simulink model "gm_DVBS"  (R2023b)
settings: Solver=FixedStepAuto  StartTime=0.0  StopTime=1  RelTol=1e-3
undefined symbols (not defined in the file or in its folder): alpha, fc, iniStates, rb
libraries: simulink x29, dspsrcs4 x4, commcnvcod2 x2, commsink2 x2, commdigbbndpm3 x2, commfilt2 x2, commhdlblkcod x2, hdlsllib x2, commcnvintrlv2 x1, dspsigops x1
settings Model: Creator=31651  LastModifiedBy=31651
settings SolverCC: AutoInsertRateTranBlk=on
settings OptimizationCC: BlockReduction=off  ConditionallyExecuteInputs=off  DefaultUnderspecifiedDataType=single  EnhancedBackFolding=on  PassReuseOutputArgsAs=Individual arguments  ZeroExternalMemoryAtStartup=off  ZeroInternalMemoryAtStartup=off  MaxStackSize=64  OptimizeBlockOrder=speed  DifferentSizesBufferReuse=on  OptimizationCustomize=off  EfficientTunableParamExpr=on
settings DebuggingCC: InheritedTsInSrcMsg=none  SingleTaskRateTransMsg=error  ParameterTunabilityLossMsg=error
settings HardwareCC: ProdBitPerPointer=32  ProdBitPerSizeT=32  ProdBitPerPtrDiffT=32  ProdLargestAtomicFloat=None  ProdIntDivRoundTo=Undefined  ProdEndianess=Unspecified  ProdWordSize=32  ProdHWDeviceType=ASIC/FPGA->ASIC/FPGA  TargetBitPerPointer=64  TargetBitPerSizeT=64  TargetBitPerPtrDiffT=64  TargetLongLongMode=on  TargetIntDivRoundTo=Zero  TargetEndianess=LittleEndian  TargetWordSize=64  TargetHWDeviceType=Custom Processor->MATLAB Host Computer  ProdEqTarget=off  HardwareBoardFeatureSet=SoCBlockset
settings SFSimCC: MATLABDynamicMemAlloc=off
settings RTWCC: Description=Embedded Coder  SystemTargetFile=ert.tlc  HardwareBoard=Xilinx Kintex-7 KC705 development board  TemplateMakefile=ert_default_tmf
settings CodeAppCC: ForceParamTrailComments=on  IgnoreCustomStorageClasses=off  OperatorAnnotations=on  SimulinkDataObjDesc=on  SFDataObjDesc=on  InsertBlockDesc=on

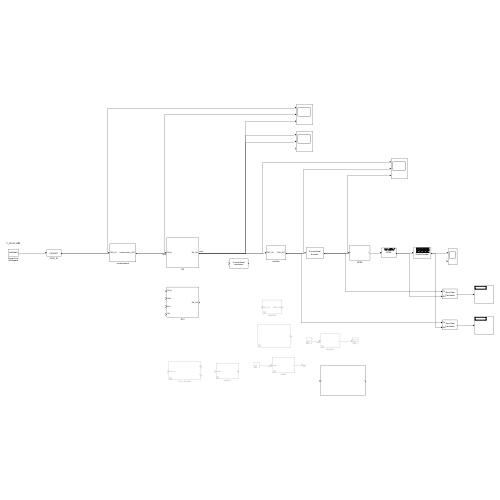
[thumbnail: Simulink's stored preview of the top-level diagram]
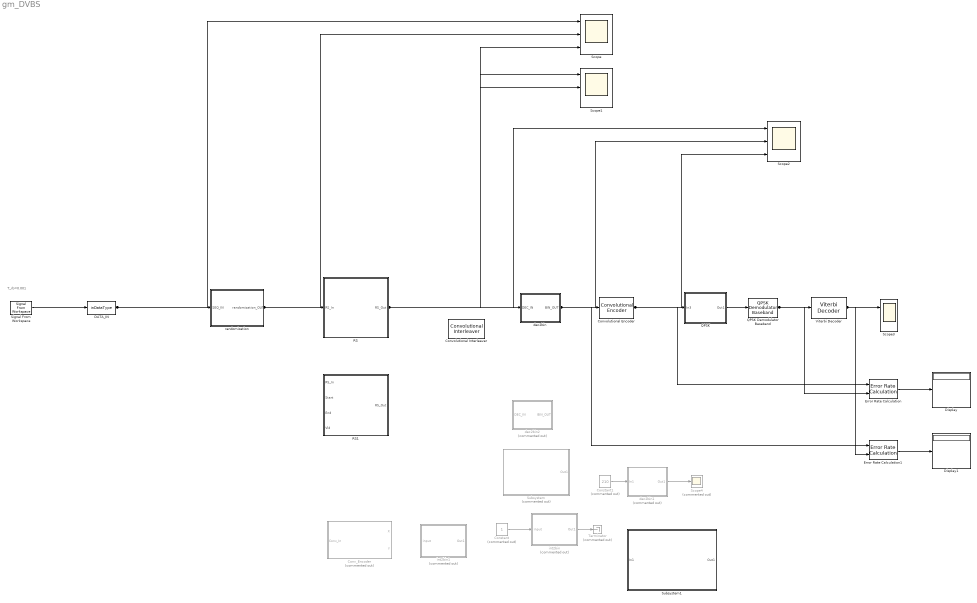
== system gm_DVBS ==
  note: T_rb=0.001
  " randomization" : Subsystem
  Constant : Constant  Commented=on  OutDataTypeStr=uint8  SampleTime=1
  Constant1 : Constant  Commented=on  Value=210  OutDataTypeStr=uint8  SampleTime=1/rb
  Conv_Encoder : Subsystem  Commented=on
  Convolutional Encoder : commcnvcod2/Convolutional Encoder  trellis=poly2trellis(7, [171 133])  opMode=Continuous  DelayedResetAction=on  hasIniStPort=off  hasFinStPort=off  usePuncVector=off  punctureVector=[1;1;0;1;1;0]  reset=Unused parameter value
      settings: LibrarySourceBlock=|
      | commhdlcnvcod/Convolutional
      | Encoder
  Convolutional Interleaver : commcnvintrlv2/Convolutional Interleaver  N=12  B=17  ic=0
      settings: LibrarySourceBlock=|
      | commhdlinterleave/Convolutional
      | Interleaver
  DATA_IN : DataTypeConversion  OutDataTypeStr=inDataType  SaturateOnIntegerOverflow=off  RndMeth=Floor
  Display : Display
  Display1 : Display
  Error Rate Calculation : commsink2/Error Rate Calculation  N=0  st_delay=0  cp_mode=Entire frame  subframe=[]  PMode=Port  WsName=ErrorVec  RsMode2=off  stop=off  numErr=100  maxBits=1e6
      settings: LibrarySourceBlock=|
      | commhdlsink/Error Rate
      | Calculation
  Error Rate Calculation1 : commsink2/Error Rate Calculation  N=64  st_delay=0  cp_mode=Entire frame  subframe=[]  PMode=Port  WsName=ErrorVec  RsMode2=off  stop=off  numErr=100  maxBits=1e6
      settings: LibrarySourceBlock=|
      | commhdlsink/Error Rate
      | Calculation
  QPSK : Subsystem
  QPSK Demodulator Baseband : commdigbbndpm3/QPSK Demodulator Baseband  OutType=Bit  DecType=Hard decision  VarSource=Dialog  Variance=1  Dec=Binary  Ph=pi/4  outDtype1=double  outDtype2=Inherit via internal rule  derotateFactorWordLen=16  derotateFactorDataTypeStr=Inherit: Same word length as input  derotateFactorLastDataTypeStr=Inherit: Same word length as input
      settings: LibrarySourceBlock=|
      | commhdldigbbndpm/QPSK
      | Demodulator
      | Baseband
  RS : Subsystem
  RS1 : Subsystem
  Scope : Scope  NumInputPorts=3
  Scope1 : Scope  NumInputPorts=3
  Scope2 : Scope  NumInputPorts=3
  Scope3 : Scope  NumInputPorts=2
  Scope4 : Scope  Commented=on
  Signal From Workspace : dspsrcs4/Signal From Workspace  X=simDataIn  Ts=1/rb  nsamps=1  OutputAfterFinalValue=Setting to zero  ignoreOrWarnInputAndFrameLengths=off  OutputFrames=off
  Subsystem : Subsystem  Commented=on
  Subsystem1 : Subsystem
  Terminator : Terminator  Commented=on
  Viterbi Decoder : commcnvcod2/Viterbi Decoder  trellis=poly2trellis(7, [171 133])  isPunctured=off  punctureVector=[1; 1; 0; 1; 0; 1]  erasures=off  dectype=Unquantized  nsdecb=4  runSigValErrCheck=off  tbdepth=64  opmode=Continuous  reset=off  delayedResetAction=off  smWordLength=16  outDataType=Inherit via internal rule
  dec2bin : Subsystem
  dec2bin1 : Subsystem  Commented=on
  dec2bin2 : Subsystem  Commented=on
  int2bin : Subsystem  Commented=on
  int2bin1 : Subsystem  Commented=on
  wires:
  Error Rate Calculation1/1 -> Display1/1
  Error Rate Calculation/1 -> Display/1
  QPSK Demodulator Baseband/1 -> Viterbi Decoder/1, Error Rate Calculation/2
  dec2bin/1(BIN_OUT) -> Scope2/2, Convolutional Encoder/1, Error Rate Calculation1/1
  QPSK/1(Out1) -> QPSK Demodulator Baseband/1
  RS/1(RS_Out) -> Scope1/1, dec2bin/1(DEC_IN), Scope1/2, Scope2/1, Scope/3
  dec2bin1/1(Out1) -> Scope4/1
  Constant1/1 -> dec2bin1/1(In1)
  Viterbi Decoder/1 -> Scope3/1, Error Rate Calculation1/2
  Convolutional Encoder/1 -> Scope2/3, QPSK/1(In3), Error Rate Calculation/1
  int2bin/1(Out1) -> Terminator/1
  Constant/1 -> int2bin/1(input)
  Signal From Workspace/1 -> DATA_IN/1
  " randomization"/1(" randomization_OUT") -> Scope/2, RS/1(RS_In)
  DATA_IN/1 -> Scope/1, " randomization"/1(SEQ_IN)

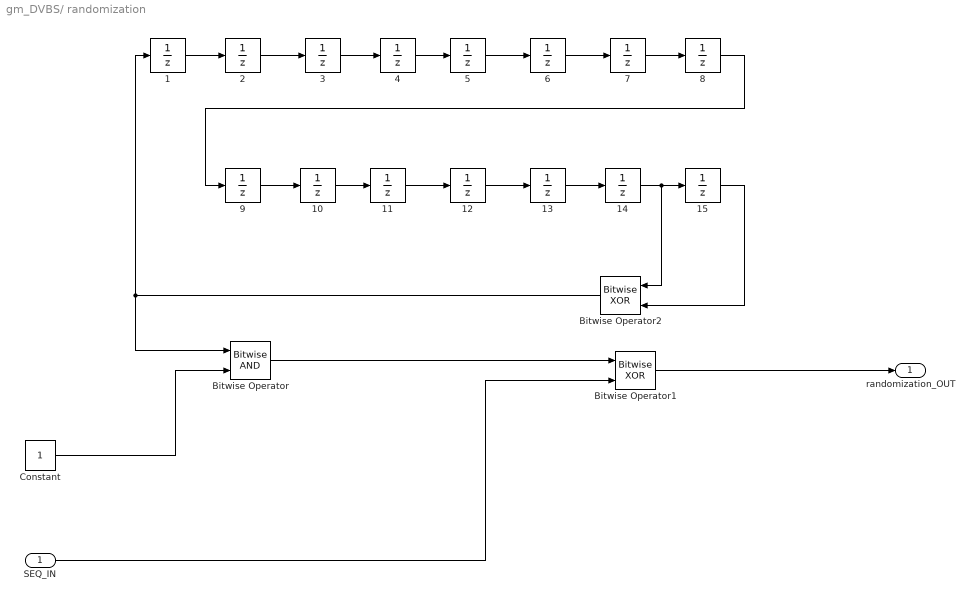
== system gm_DVBS/ randomization ==
  SEQ_IN : Inport
  1 : UnitDelay  InitialCondition=iniStates(1)  SampleTime=1/rb  HasFrameUpgradeWarning=on
  10 : UnitDelay  InitialCondition=iniStates(10)  SampleTime=-1  HasFrameUpgradeWarning=on
  11 : UnitDelay  InitialCondition=iniStates(11)  SampleTime=-1  HasFrameUpgradeWarning=on
  12 : UnitDelay  InitialCondition=iniStates(12)  SampleTime=-1  HasFrameUpgradeWarning=on
  13 : UnitDelay  InitialCondition=iniStates(13)  SampleTime=-1  HasFrameUpgradeWarning=on
  14 : UnitDelay  InitialCondition=iniStates(14)  SampleTime=-1  HasFrameUpgradeWarning=on
  15 : UnitDelay  InitialCondition=iniStates(15)  SampleTime=-1  HasFrameUpgradeWarning=on
  2 : UnitDelay  InitialCondition=iniStates(2)  SampleTime=-1  HasFrameUpgradeWarning=on
  3 : UnitDelay  InitialCondition=iniStates(3)  SampleTime=-1  HasFrameUpgradeWarning=on
  4 : UnitDelay  InitialCondition=iniStates(4)  SampleTime=-1  HasFrameUpgradeWarning=on
  5 : UnitDelay  InitialCondition=iniStates(5)  SampleTime=-1  HasFrameUpgradeWarning=on
  6 : UnitDelay  InitialCondition=iniStates(6)  SampleTime=-1  HasFrameUpgradeWarning=on
  7 : UnitDelay  InitialCondition=iniStates(7)  SampleTime=-1  HasFrameUpgradeWarning=on
  8 : UnitDelay  InitialCondition=iniStates(8)  SampleTime=-1  HasFrameUpgradeWarning=on
  9 : UnitDelay  InitialCondition=iniStates(9)  SampleTime=-1  HasFrameUpgradeWarning=on
  Bitwise Operator : simulink/Logic and Bit Operations/Bitwise Operator  logicop=AND  UseBitMask=off  NumInputPorts=2  BitMask=bin2dec('11011001')  BitMaskRealWorld=Stored Integer
      settings: LibrarySourceBlock=|
      | hdlsllib/Logic and Bit
      | Operations/Bitwise
      | Operator
  Bitwise Operator1 : simulink/Logic and Bit Operations/Bitwise Operator  logicop=XOR  UseBitMask=off  NumInputPorts=2  BitMask=bin2dec('11011001')  BitMaskRealWorld=Stored Integer
      settings: LibrarySourceBlock=|
      | hdlsllib/Logic and Bit
      | Operations/Bitwise
      | Operator
  Bitwise Operator2 : simulink/Logic and Bit Operations/Bitwise Operator  logicop=XOR  UseBitMask=off  NumInputPorts=2  BitMask=bin2dec('11011001')  BitMaskRealWorld=Stored Integer
      settings: LibrarySourceBlock=|
      | hdlsllib/Logic and Bit
      | Operations/Bitwise
      | Operator
  Constant : Constant  OutDataTypeStr=inDataType  SampleTime=1/rb
  " randomization_OUT" : Outport
  wires:
  Bitwise Operator1/1 -> " randomization_OUT"/1
  SEQ_IN/1 -> Bitwise Operator1/2
  Constant/1 -> Bitwise Operator/2
  Bitwise Operator/1 -> Bitwise Operator1/1
  Bitwise Operator2/1 -> 1/1, Bitwise Operator/1
  15/1 -> Bitwise Operator2/2
  12/1 -> 13/1
  13/1 -> 14/1
  14/1 -> 15/1, Bitwise Operator2/1
  6/1 -> 7/1
  7/1 -> 8/1
  11/1 -> 12/1
  8/1 -> 9/1
  10/1 -> 11/1
  9/1 -> 10/1
  1/1 -> 2/1
  3/1 -> 4/1
  2/1 -> 3/1
  4/1 -> 5/1
  5/1 -> 6/1

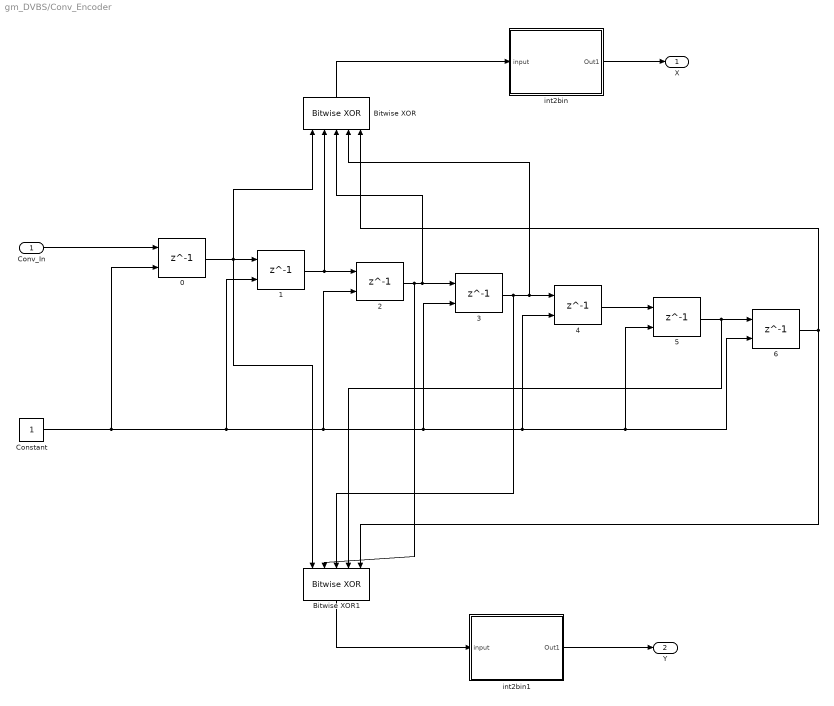
== system gm_DVBS/Conv_Encoder ==
  Conv_In : Inport
  {0..6} (7 alike) : Delay  DelayLength=1  ShowEnablePort=on
      settings: InputPortMap=u0,e6
  Bitwise XOR : simulink/Logic and Bit Operations/Bitwise Operator  logicop=XOR  UseBitMask=off  NumInputPorts=5  BitMask=bin2dec('11011001')  BitMaskRealWorld=Stored Integer
      settings: LibrarySourceBlock=|
      | simulink/Quick Insert/Logic and Bit
      | Operations/Bitwise XOR
  Bitwise XOR1 : simulink/Logic and Bit Operations/Bitwise Operator  logicop=XOR  UseBitMask=off  NumInputPorts=5  BitMask=bin2dec('11011001')  BitMaskRealWorld=Stored Integer
      settings: LibrarySourceBlock=|
      | simulink/Quick Insert/Logic and Bit
      | Operations/Bitwise XOR
  Constant : Constant  OutDataTypeStr=boolean  SampleTime=1/rb
  int2bin : Subsystem
  int2bin1 : Subsystem
  X : Outport
  Y : Outport  Port=2
  wires:
  int2bin1/1(Out1) -> Y/1
  Bitwise XOR/1 -> int2bin/1(input)
  int2bin/1(Out1) -> X/1
  Bitwise XOR1/1 -> int2bin1/1(input)
  6/1 -> Bitwise XOR/5, Bitwise XOR1/5
  Constant/1 -> 6/2, 5/2, 4/2, 3/2, 2/2, 1/2, 0/2
  Conv_In/1 -> 0/1
  0/1 -> 1/1, Bitwise XOR/1, Bitwise XOR1/1
  1/1 -> 2/1, Bitwise XOR/2
  2/1 -> 3/1, Bitwise XOR/3, Bitwise XOR1/2
  3/1 -> 4/1, Bitwise XOR/4, Bitwise XOR1/3
  4/1 -> 5/1
  5/1 -> 6/1, Bitwise XOR1/4

== system gm_DVBS/QPSK ==
  In3 : Inport
  Add : Sum
  Complex to Real-Imag : ComplexToRealImag
  Cos : Sin  Frequency=fc*2*pi  Phase=pi/2  SampleTime=0
  Product : Product
  Product1 : Product
  QPSK Modulator Baseband : commdigbbndpm3/QPSK Modulator Baseband  InType=Bit  Enc=Binary  Ph=pi/4  outDtype=double  outWordLen=16  outUDDataType=sfix(16)  outFracLenMode=Best precision  outFracLen=15  outDataTypeStr=double  outLastDataTypeStr=double
      settings: LibrarySourceBlock=|
      | commhdldigbbndpm/QPSK
      | Modulator
      | Baseband
  Raised Cosine Transmit Filter2 : commfilt2/Raised Cosine Transmit Filter  filtType=Square root  R=alpha  filtSpan=10  N=8  filterGain=1  InputProcessing=Columns as channels (frame based)  RateOptions=Allow multirate processing  framing=Mute  checkCoeff=off  variableName=rcTxFilt2  checkGain=Normalized  sampMode=Mute  saveAsFlag=0  currentFiltSpan=10  D=5  launchFVT=on  roundingMode=Floor  overflowMode=off  coeffDataTypeStr=Inherit: Same word length as input  coeffMin=[]  coeffMax=[]  coeffLastDataTypeStr=Inherit: Same word length as input  outputDataTypeStr=Inherit: Same as accumulator  outputMin=[]  outputMax=[]  outputLastDataTypeStr=Inherit: Same as accumulator
      settings: LibrarySourceBlock=|
      | commhdlfilt/Raised Cosine
      | Transmit Filter
  Raised Cosine Transmit Filter3 : commfilt2/Raised Cosine Transmit Filter  filtType=Square root  R=alpha  filtSpan=10  N=8  filterGain=1  RateOptions=Allow multirate processing  framing=Mute  checkCoeff=off  variableName=rcTxFilt3  checkGain=Normalized  sampMode=Mute  saveAsFlag=0  currentFiltSpan=10  D=5  launchFVT=on  roundingMode=Floor  overflowMode=off  coeffDataTypeStr=Inherit: Same word length as input  coeffMin=[]  coeffMax=[]  coeffLastDataTypeStr=Inherit: Same word length as input  outputDataTypeStr=Inherit: Same as accumulator  outputMin=[]  outputMax=[]  outputLastDataTypeStr=Inherit: Same as accumulator
      settings: LibrarySourceBlock=|
      | commhdlfilt/Raised Cosine
      | Transmit Filter
  Scope : Scope
  Scope1 : Scope  NumInputPorts=2
  Sin : Sin  Frequency=fc*2*pi  SampleTime=0
  Spectrum Analyzer : SpectrumAnalyzer  WindowPosition=[560.000000,290.000000,800.000000,500.000000,]  ScopeFrameLocation=window  Span=24000  StartFrequency=-12000  StopFrequency=12000  YLimits=[-206.50491474,-40.69069962]
      settings: OpenAtSimulationStart=off
  Zero-Order Hold : ZeroOrderHold  SampleTime=-1
  Out1 : Outport
  wires:
  Zero-Order Hold/1 -> Spectrum Analyzer/1
  Add/1 -> Zero-Order Hold/1, Scope/1
  Product1/1 -> Add/2
  Complex to Real-Imag/2 -> Raised Cosine Transmit Filter3/1
  Cos/1 -> Product/2, Scope1/2
  Sin/1 -> Product1/1
  Complex to Real-Imag/1 -> Raised Cosine Transmit Filter2/1
  Raised Cosine Transmit Filter2/1 -> Product/1
  Raised Cosine Transmit Filter3/1 -> Product1/2
  Product/1 -> Add/1, Scope1/1
  In3/1 -> QPSK Modulator Baseband/1
  QPSK Modulator Baseband/1 -> Complex to Real-Imag/1, Out1/1

== system gm_DVBS/RS ==
  RS_In : Inport  OutDataTypeStr=uint8
  Data Type Conversion : DataTypeConversion  OutDataTypeStr=boolean  SaturateOnIntegerOverflow=off  RndMeth=Floor
  Data Type Conversion1 : DataTypeConversion  OutDataTypeStr=boolean  SaturateOnIntegerOverflow=off  RndMeth=Floor
  Data Type Conversion2 : DataTypeConversion  OutDataTypeStr=boolean  SaturateOnIntegerOverflow=off  RndMeth=Floor
  Integer-Input RS Encoder HDL Optimized : commhdlblkcod/Integer-Input RS Encoder HDL Optimized  CodewordLength=n  MessageLength=k  PrimitivePolynomialSource=Auto  PrimitivePolynomial=[ 1, 0, 1, 1 ]  PuncturePatternSource=None  PuncturePattern=[ ones( 2, 1 ); zeros( 2, 1 ) ]  BSource=Auto  B=1  SimulateUsing=Code generation
  Signal From Workspace1 : dspsrcs4/Signal From Workspace  X=simStart  Ts=1/rb  nsamps=1  OutputAfterFinalValue=Setting to zero  ignoreOrWarnInputAndFrameLengths=off  OutputFrames=off
  Signal From Workspace2 : dspsrcs4/Signal From Workspace  X=simEnd  Ts=1/rb  nsamps=1  OutputAfterFinalValue=Setting to zero  ignoreOrWarnInputAndFrameLengths=off  OutputFrames=off
  Signal From Workspace3 : dspsrcs4/Signal From Workspace  X=simValidIn  Ts=1/rb  nsamps=1  OutputAfterFinalValue=Setting to zero  ignoreOrWarnInputAndFrameLengths=off  OutputFrames=off
  RS_Out : Outport  OutDataTypeStr=uint8
  wires:
  Integer-Input RS Encoder HDL Optimized/1 -> RS_Out/1
  RS_In/1 -> Integer-Input RS Encoder HDL Optimized/1
  Data Type Conversion2/1 -> Integer-Input RS Encoder HDL Optimized/4
  Signal From Workspace1/1 -> Data Type Conversion/1
  Signal From Workspace2/1 -> Data Type Conversion1/1
  Signal From Workspace3/1 -> Data Type Conversion2/1
  Data Type Conversion1/1 -> Integer-Input RS Encoder HDL Optimized/3
  Data Type Conversion/1 -> Integer-Input RS Encoder HDL Optimized/2

== system gm_DVBS/RS1 ==
  RS_In : Inport  OutDataTypeStr=uint8
  Start : Inport  Port=2
  End : Inport  Port=3
  Vld : Inport  Port=4
  Data Type Conversion : DataTypeConversion  OutDataTypeStr=boolean  SaturateOnIntegerOverflow=off  RndMeth=Floor
  Data Type Conversion1 : DataTypeConversion  OutDataTypeStr=boolean  SaturateOnIntegerOverflow=off  RndMeth=Floor
  Data Type Conversion2 : DataTypeConversion  OutDataTypeStr=boolean  SaturateOnIntegerOverflow=off  RndMeth=Floor
  Integer-Input RS Encoder HDL Optimized : commhdlblkcod/Integer-Input RS Encoder HDL Optimized  CodewordLength=n  MessageLength=k  PrimitivePolynomialSource=Auto  PrimitivePolynomial=[ 1, 0, 1, 1 ]  PuncturePatternSource=None  PuncturePattern=[ ones( 2, 1 ); zeros( 2, 1 ) ]  BSource=Auto  B=1  SimulateUsing=Code generation
  Terminator : Terminator
  Terminator1 : Terminator
  Terminator2 : Terminator
  RS_Out : Outport  OutDataTypeStr=uint8
  wires:
  Integer-Input RS Encoder HDL Optimized/4 -> Terminator2/1
  Integer-Input RS Encoder HDL Optimized/3 -> Terminator1/1
  Integer-Input RS Encoder HDL Optimized/2 -> Terminator/1
  Vld/1 -> Data Type Conversion2/1
  End/1 -> Data Type Conversion1/1
  Start/1 -> Data Type Conversion/1
  Integer-Input RS Encoder HDL Optimized/1 -> RS_Out/1
  RS_In/1 -> Integer-Input RS Encoder HDL Optimized/1
  Data Type Conversion2/1 -> Integer-Input RS Encoder HDL Optimized/4
  Data Type Conversion1/1 -> Integer-Input RS Encoder HDL Optimized/3
  Data Type Conversion/1 -> Integer-Input RS Encoder HDL Optimized/2

== system gm_DVBS/Subsystem ==
  Constant1 : Constant  Value=113  SampleTime=1
  Demux : Demux  Outputs=8
      settings: DisplayOption=none
  MATLAB Function : MATLAB Function  TreatAsAtomicUnit=on
  Scope : Scope
  Subsystem1 : Subsystem
  Out1 : Outport
  wires:
  Subsystem1/1(Out1) -> Out1/1, Scope/1
  MATLAB Function/1(bin_out) -> Demux/1
  Demux/8 -> Subsystem1/8(In8)
  Demux/7 -> Subsystem1/7(In7)
  Demux/6 -> Subsystem1/6(In6)
  Demux/5 -> Subsystem1/5(In5)
  Demux/4 -> Subsystem1/4(In4)
  Demux/3 -> Subsystem1/3(In3)
  Demux/2 -> Subsystem1/2(In2)
  Demux/1 -> Subsystem1/1(In1)
  Constant1/1 -> MATLAB Function/1(dec_in)

== system gm_DVBS/Subsystem1 ==
  In1 : Inport
  Out1 : Outport
  wires:
  In1/1 -> Out1/1

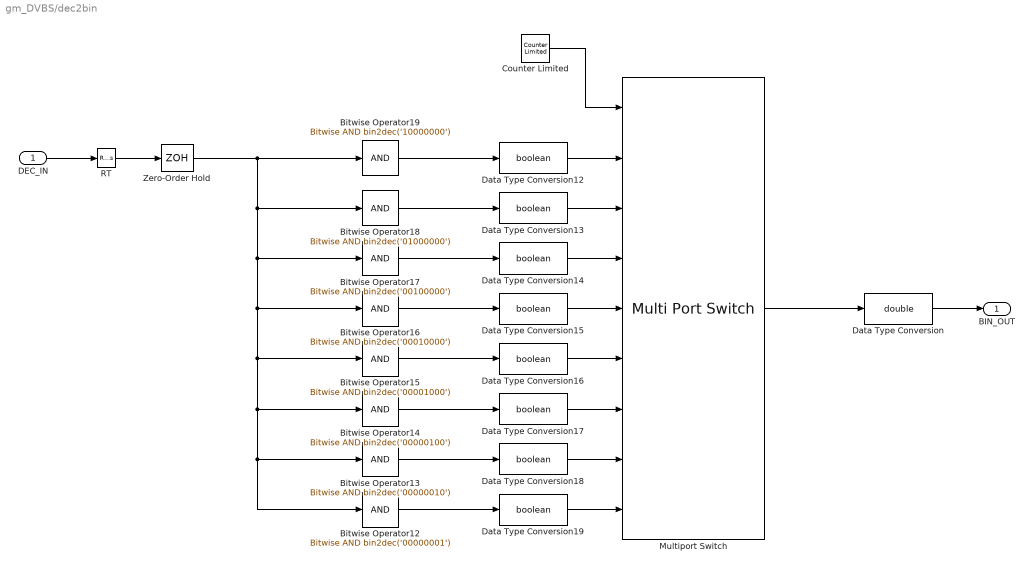
== system gm_DVBS/dec2bin ==
  DEC_IN : Inport
  Bitwise Operator12 : simulink/Logic and Bit Operations/Bitwise Operator  logicop=AND  UseBitMask=on  BitMask=bin2dec('00000001')  BitMaskRealWorld=Stored Integer
  Bitwise Operator13 : simulink/Logic and Bit Operations/Bitwise Operator  logicop=AND  UseBitMask=on  BitMask=bin2dec('00000010')  BitMaskRealWorld=Stored Integer
  Bitwise Operator14 : simulink/Logic and Bit Operations/Bitwise Operator  logicop=AND  UseBitMask=on  BitMask=bin2dec('00000100')  BitMaskRealWorld=Stored Integer
  Bitwise Operator15 : simulink/Logic and Bit Operations/Bitwise Operator  logicop=AND  UseBitMask=on  BitMask=bin2dec('00001000')  BitMaskRealWorld=Stored Integer
  Bitwise Operator16 : simulink/Logic and Bit Operations/Bitwise Operator  logicop=AND  UseBitMask=on  BitMask=bin2dec('00010000')  BitMaskRealWorld=Stored Integer
  Bitwise Operator17 : simulink/Logic and Bit Operations/Bitwise Operator  logicop=AND  UseBitMask=on  BitMask=bin2dec('00100000')  BitMaskRealWorld=Stored Integer
  Bitwise Operator18 : simulink/Logic and Bit Operations/Bitwise Operator  logicop=AND  UseBitMask=on  BitMask=bin2dec('01000000')  BitMaskRealWorld=Stored Integer
  Bitwise Operator19 : simulink/Logic and Bit Operations/Bitwise Operator  logicop=AND  UseBitMask=on  BitMask=bin2dec('10000000')  BitMaskRealWorld=Stored Integer
  Counter Limited : hdlsllib/Sources/Counter Limited  uplimit=7  tsamp=0.125/rb
  Data Type Conversion : DataTypeConversion  OutDataTypeStr=double  SaturateOnIntegerOverflow=off  RndMeth=Floor
  Data Type Conversion{12..19} (8 alike) : DataTypeConversion  OutDataTypeStr=boolean  SaturateOnIntegerOverflow=off  RndMeth=Floor
  Multiport Switch : MultiPortSwitch  DataPortOrder=Zero-based contiguous  Inputs=8  zeroidx=on  SaturateOnIntegerOverflow=off  InputSameDT=off
  RT : RateTransition  OutPortSampleTime=0.000125
  Zero-Order Hold : ZeroOrderHold  SampleTime=0.125/rb
  BIN_OUT : Outport
  wires:
  Data Type Conversion/1 -> BIN_OUT/1
  Multiport Switch/1 -> Data Type Conversion/1
  RT/1 -> Zero-Order Hold/1
  Zero-Order Hold/1 -> Bitwise Operator17/1, Bitwise Operator14/1, Bitwise Operator12/1, Bitwise Operator13/1, Bitwise Operator15/1, Bitwise Operator16/1, Bitwise Operator18/1, Bitwise Operator19/1
  Bitwise Operator17/1 -> Data Type Conversion14/1
  Data Type Conversion19/1 -> Multiport Switch/9
  Data Type Conversion17/1 -> Multiport Switch/7
  Data Type Conversion13/1 -> Multiport Switch/3
  Bitwise Operator12/1 -> Data Type Conversion19/1
  Data Type Conversion16/1 -> Multiport Switch/6
  Data Type Conversion15/1 -> Multiport Switch/5
  Data Type Conversion14/1 -> Multiport Switch/4
  Data Type Conversion18/1 -> Multiport Switch/8
  Data Type Conversion12/1 -> Multiport Switch/2
  Bitwise Operator16/1 -> Data Type Conversion15/1
  Counter Limited/1 -> Multiport Switch/1
  DEC_IN/1 -> RT/1
  Bitwise Operator14/1 -> Data Type Conversion17/1
  Bitwise Operator15/1 -> Data Type Conversion16/1
  Bitwise Operator19/1 -> Data Type Conversion12/1
  Bitwise Operator18/1 -> Data Type Conversion13/1
  Bitwise Operator13/1 -> Data Type Conversion18/1

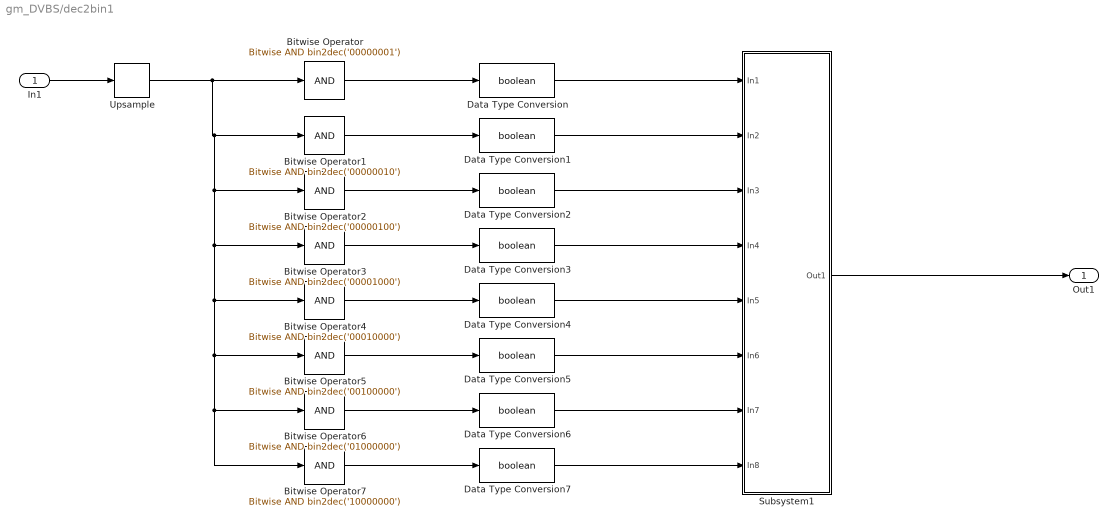
== system gm_DVBS/dec2bin1 ==
  In1 : Inport  OutDataTypeStr=uint8
  Bitwise Operator : simulink/Logic and Bit Operations/Bitwise Operator  logicop=AND  UseBitMask=on  BitMask=bin2dec('00000001')  BitMaskRealWorld=Stored Integer
  Bitwise Operator1 : simulink/Logic and Bit Operations/Bitwise Operator  logicop=AND  UseBitMask=on  BitMask=bin2dec('00000010')  BitMaskRealWorld=Stored Integer
  Bitwise Operator2 : simulink/Logic and Bit Operations/Bitwise Operator  logicop=AND  UseBitMask=on  BitMask=bin2dec('00000100')  BitMaskRealWorld=Stored Integer
  Bitwise Operator3 : simulink/Logic and Bit Operations/Bitwise Operator  logicop=AND  UseBitMask=on  BitMask=bin2dec('00001000')  BitMaskRealWorld=Stored Integer
  Bitwise Operator4 : simulink/Logic and Bit Operations/Bitwise Operator  logicop=AND  UseBitMask=on  BitMask=bin2dec('00010000')  BitMaskRealWorld=Stored Integer
  Bitwise Operator5 : simulink/Logic and Bit Operations/Bitwise Operator  logicop=AND  UseBitMask=on  BitMask=bin2dec('00100000')  BitMaskRealWorld=Stored Integer
  Bitwise Operator6 : simulink/Logic and Bit Operations/Bitwise Operator  logicop=AND  UseBitMask=on  BitMask=bin2dec('01000000')  BitMaskRealWorld=Stored Integer
  Bitwise Operator7 : simulink/Logic and Bit Operations/Bitwise Operator  logicop=AND  UseBitMask=on  BitMask=bin2dec('10000000')  BitMaskRealWorld=Stored Integer
  Data Type Conversion{,1..7} (8 alike) : DataTypeConversion  OutDataTypeStr=boolean  SaturateOnIntegerOverflow=off  RndMeth=Floor
  Subsystem1 : Subsystem
  Upsample : dspsigops/Upsample  FactorSource=Dialog parameter  N=3  Nmax=16  phase=0  RateOptions=Allow multirate processing  ic=0  mode=Unused parameter value
      settings: LibrarySourceBlock=dsphdlsupportsigops/Upsample
  Out1 : Outport
  wires:
  Upsample/1 -> Bitwise Operator/1, Bitwise Operator1/1, Bitwise Operator2/1, Bitwise Operator3/1, Bitwise Operator4/1, Bitwise Operator5/1, Bitwise Operator6/1, Bitwise Operator7/1
  Bitwise Operator/1 -> Data Type Conversion/1
  Bitwise Operator1/1 -> Data Type Conversion1/1
  Bitwise Operator3/1 -> Data Type Conversion3/1
  Bitwise Operator4/1 -> Data Type Conversion4/1
  Bitwise Operator2/1 -> Data Type Conversion2/1
  Data Type Conversion2/1 -> Subsystem1/3(In3)
  Bitwise Operator5/1 -> Data Type Conversion5/1
  Bitwise Operator6/1 -> Data Type Conversion6/1
  Bitwise Operator7/1 -> Data Type Conversion7/1
  In1/1 -> Upsample/1
  Data Type Conversion3/1 -> Subsystem1/4(In4)
  Subsystem1/1(Out1) -> Out1/1
  Data Type Conversion6/1 -> Subsystem1/7(In7)
  Data Type Conversion1/1 -> Subsystem1/2(In2)
  Data Type Conversion7/1 -> Subsystem1/8(In8)
  Data Type Conversion5/1 -> Subsystem1/6(In6)
  Data Type Conversion/1 -> Subsystem1/1(In1)
  Data Type Conversion4/1 -> Subsystem1/5(In5)

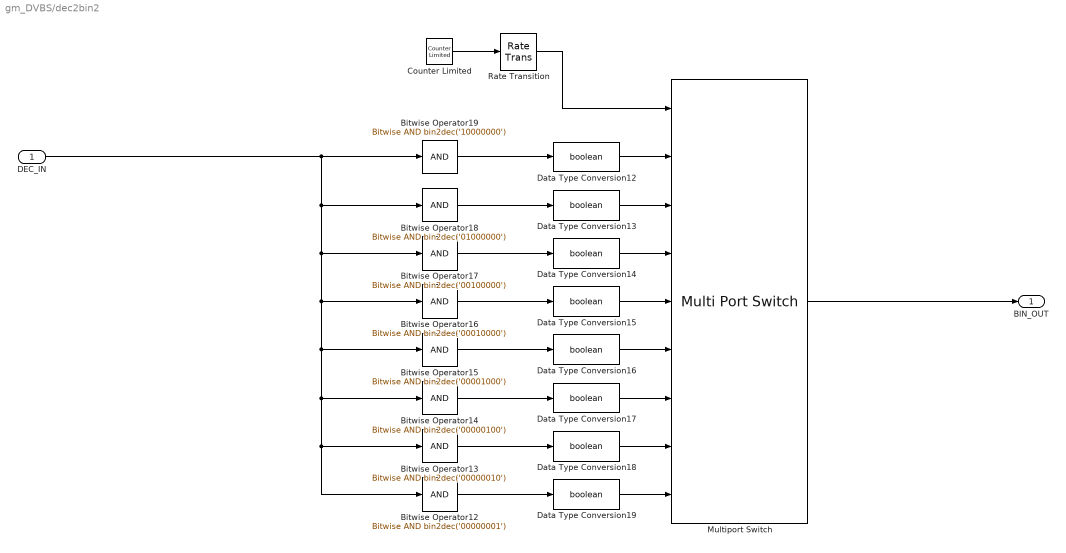
== system gm_DVBS/dec2bin2 ==
  DEC_IN : Inport  OutDataTypeStr=uint8
  Bitwise Operator12 : simulink/Logic and Bit Operations/Bitwise Operator  logicop=AND  UseBitMask=on  BitMask=bin2dec('00000001')  BitMaskRealWorld=Stored Integer
  Bitwise Operator13 : simulink/Logic and Bit Operations/Bitwise Operator  logicop=AND  UseBitMask=on  BitMask=bin2dec('00000010')  BitMaskRealWorld=Stored Integer
  Bitwise Operator14 : simulink/Logic and Bit Operations/Bitwise Operator  logicop=AND  UseBitMask=on  BitMask=bin2dec('00000100')  BitMaskRealWorld=Stored Integer
  Bitwise Operator15 : simulink/Logic and Bit Operations/Bitwise Operator  logicop=AND  UseBitMask=on  BitMask=bin2dec('00001000')  BitMaskRealWorld=Stored Integer
  Bitwise Operator16 : simulink/Logic and Bit Operations/Bitwise Operator  logicop=AND  UseBitMask=on  BitMask=bin2dec('00010000')  BitMaskRealWorld=Stored Integer
  Bitwise Operator17 : simulink/Logic and Bit Operations/Bitwise Operator  logicop=AND  UseBitMask=on  BitMask=bin2dec('00100000')  BitMaskRealWorld=Stored Integer
  Bitwise Operator18 : simulink/Logic and Bit Operations/Bitwise Operator  logicop=AND  UseBitMask=on  BitMask=bin2dec('01000000')  BitMaskRealWorld=Stored Integer
  Bitwise Operator19 : simulink/Logic and Bit Operations/Bitwise Operator  logicop=AND  UseBitMask=on  BitMask=bin2dec('10000000')  BitMaskRealWorld=Stored Integer
  Counter Limited : hdlsllib/Sources/Counter Limited  uplimit=7  tsamp=0.125/rb
  Data Type Conversion{12..19} (8 alike) : DataTypeConversion  OutDataTypeStr=boolean  SaturateOnIntegerOverflow=off  RndMeth=Floor
  Multiport Switch : MultiPortSwitch  DataPortOrder=Zero-based contiguous  Inputs=8  zeroidx=on  SaturateOnIntegerOverflow=off  InputSameDT=off
  Rate Transition : RateTransition  OutPortSampleTime=0.125/rb
  BIN_OUT : Outport
  wires:
  Rate Transition/1 -> Multiport Switch/1
  DEC_IN/1 -> Bitwise Operator19/1, Bitwise Operator17/1, Bitwise Operator14/1, Bitwise Operator12/1, Bitwise Operator13/1, Bitwise Operator15/1, Bitwise Operator16/1, Bitwise Operator18/1
  Counter Limited/1 -> Rate Transition/1
  Multiport Switch/1 -> BIN_OUT/1
  Bitwise Operator17/1 -> Data Type Conversion14/1
  Data Type Conversion19/1 -> Multiport Switch/9
  Data Type Conversion17/1 -> Multiport Switch/7
  Data Type Conversion13/1 -> Multiport Switch/3
  Bitwise Operator12/1 -> Data Type Conversion19/1
  Data Type Conversion16/1 -> Multiport Switch/6
  Data Type Conversion15/1 -> Multiport Switch/5
  Data Type Conversion14/1 -> Multiport Switch/4
  Data Type Conversion18/1 -> Multiport Switch/8
  Data Type Conversion12/1 -> Multiport Switch/2
  Bitwise Operator16/1 -> Data Type Conversion15/1
  Bitwise Operator14/1 -> Data Type Conversion17/1
  Bitwise Operator15/1 -> Data Type Conversion16/1
  Bitwise Operator19/1 -> Data Type Conversion12/1
  Bitwise Operator18/1 -> Data Type Conversion13/1
  Bitwise Operator13/1 -> Data Type Conversion18/1

== system gm_DVBS/int2bin ==
  note: 最低位
  input : Inport  OutDataTypeStr=uint8
  Data Type Conversion : DataTypeConversion  OutDataTypeStr=boolean  SaturateOnIntegerOverflow=off  RndMeth=Floor
  Demux : Demux  Outputs=8
      settings: DisplayOption=none
  PISO : Subsystem
  Scope3 : Scope  NumInputPorts=4
  Scope4 : Scope  NumInputPorts=4
  uint8tobin : MATLAB Function  TreatAsAtomicUnit=on
  Out1 : Outport
  wires:
  Data Type Conversion/1 -> Demux/1
  Demux/2 -> Scope3/2, PISO/2(2)
  Demux/3 -> Scope3/3, PISO/3(3)
  Demux/4 -> Scope3/4, PISO/4(4)
  input/1 -> uint8tobin/1(input)
  Demux/7 -> Scope4/3, PISO/7(7)
  Demux/1 -> Scope3/1, PISO/1(1)
  uint8tobin/1(bitValue) -> Data Type Conversion/1
  Demux/8 -> Scope4/4, PISO/8(8)
  Demux/5 -> Scope4/1, PISO/5(5)
  Demux/6 -> Scope4/2, PISO/6(6)
  PISO/1(Out1) -> Out1/1

== system gm_DVBS/int2bin1 ==
  note: 最低位
  input : Inport  OutDataTypeStr=uint8
  Data Type Conversion : DataTypeConversion  OutDataTypeStr=boolean  SaturateOnIntegerOverflow=off  RndMeth=Floor
  Demux : Demux  Outputs=8
      settings: DisplayOption=none
  PISO : Subsystem
  Scope3 : Scope  NumInputPorts=4
  Scope4 : Scope  NumInputPorts=4
  uint8tobin : MATLAB Function  TreatAsAtomicUnit=on
  Out1 : Outport
  wires:
  Data Type Conversion/1 -> Demux/1
  Demux/2 -> Scope3/2, PISO/2(2)
  Demux/3 -> Scope3/3, PISO/3(3)
  Demux/4 -> Scope3/4, PISO/4(4)
  input/1 -> uint8tobin/1(input)
  Demux/7 -> Scope4/3, PISO/7(7)
  Demux/1 -> Scope3/1, PISO/1(1)
  uint8tobin/1(bitValue) -> Data Type Conversion/1
  Demux/8 -> Scope4/4, PISO/8(8)
  Demux/5 -> Scope4/1, PISO/5(5)
  Demux/6 -> Scope4/2, PISO/6(6)
  PISO/1(Out1) -> Out1/1

== system gm_DVBS/Conv_Encoder/int2bin ==
  note: 最低位
  input : Inport
  Demux : Demux  Outputs=8
      settings: DisplayOption=none
  PISO : Subsystem
  Scope3 : Scope  NumInputPorts=4
  Scope4 : Scope  NumInputPorts=4
  uint8tobin : MATLAB Function  TreatAsAtomicUnit=on
  Out1 : Outport
  wires:
  Demux/2 -> Scope3/2, PISO/2(2)
  Demux/3 -> Scope3/3, PISO/3(3)
  Demux/4 -> Scope3/4, PISO/4(4)
  input/1 -> uint8tobin/1(input)
  Demux/7 -> Scope4/3, PISO/7(7)
  Demux/1 -> Scope3/1, PISO/1(1)
  uint8tobin/1(bitValue) -> Demux/1
  Demux/8 -> Scope4/4, PISO/8(8)
  Demux/5 -> Scope4/1, PISO/5(5)
  Demux/6 -> Scope4/2, PISO/6(6)
  PISO/1(Out1) -> Out1/1

== system gm_DVBS/Conv_Encoder/int2bin1 ==
  note: 最低位
  input : Inport
  Demux : Demux  Outputs=8
      settings: DisplayOption=none
  PISO : Subsystem
  Scope3 : Scope  NumInputPorts=4
  Scope4 : Scope  NumInputPorts=4
  uint8tobin : MATLAB Function  TreatAsAtomicUnit=on
  Out1 : Outport
  wires:
  Demux/2 -> Scope3/2, PISO/2(2)
  Demux/3 -> Scope3/3, PISO/3(3)
  Demux/4 -> Scope3/4, PISO/4(4)
  input/1 -> uint8tobin/1(input)
  Demux/7 -> Scope4/3, PISO/7(7)
  Demux/1 -> Scope3/1, PISO/1(1)
  uint8tobin/1(bitValue) -> Demux/1
  Demux/8 -> Scope4/4, PISO/8(8)
  Demux/5 -> Scope4/1, PISO/5(5)
  Demux/6 -> Scope4/2, PISO/6(6)
  PISO/1(Out1) -> Out1/1

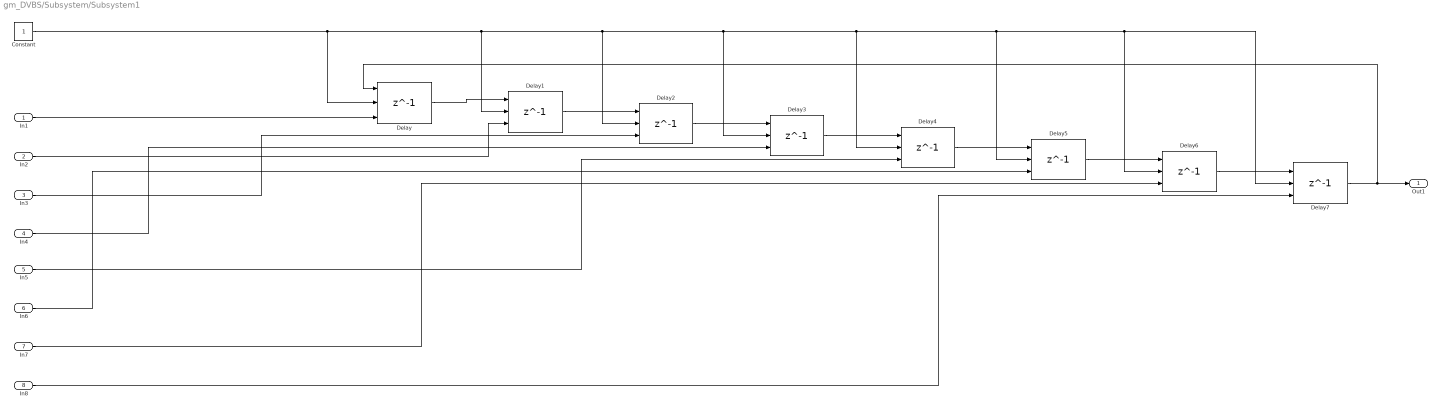
== system gm_DVBS/Subsystem/Subsystem1 ==
  In1 : Inport
  In2 : Inport  Port=2
  In3 : Inport  Port=3
  In4 : Inport  Port=4
  In5 : Inport  Port=5
  In6 : Inport  Port=6
  In7 : Inport  Port=7
  In8 : Inport  Port=8
  Constant : Constant  OutDataTypeStr=boolean  SampleTime=8
  Delay : Delay  DelayLength=1  InitialConditionSource=Input port  ExternalReset=Level hold
      settings: InputPortMap=u0,r5,p4
  Delay1 : Delay  DelayLength=1  InitialConditionSource=Input port  ExternalReset=Level hold
      settings: InputPortMap=u0,r5,p4
  Delay{2..7} (6 alike) : Delay  DelayLength=1  InitialConditionSource=Input port  ExternalReset=Rising
      settings: InputPortMap=u0,r5,p4
  Out1 : Outport
  wires:
  Constant/1 -> Delay6/2, Delay7/2, Delay5/2, Delay4/2, Delay3/2, Delay2/2, Delay1/2, Delay/2
  Delay7/1 -> Out1/1, Delay/1
  Delay3/1 -> Delay4/1
  Delay4/1 -> Delay5/1
  Delay5/1 -> Delay6/1
  Delay6/1 -> Delay7/1
  In6/1 -> Delay5/3
  In5/1 -> Delay4/3
  In8/1 -> Delay7/3
  In7/1 -> Delay6/3
  In4/1 -> Delay3/3
  In3/1 -> Delay2/3
  In2/1 -> Delay1/3
  In1/1 -> Delay/3
  Delay2/1 -> Delay3/1
  Delay1/1 -> Delay2/1
  Delay/1 -> Delay1/1

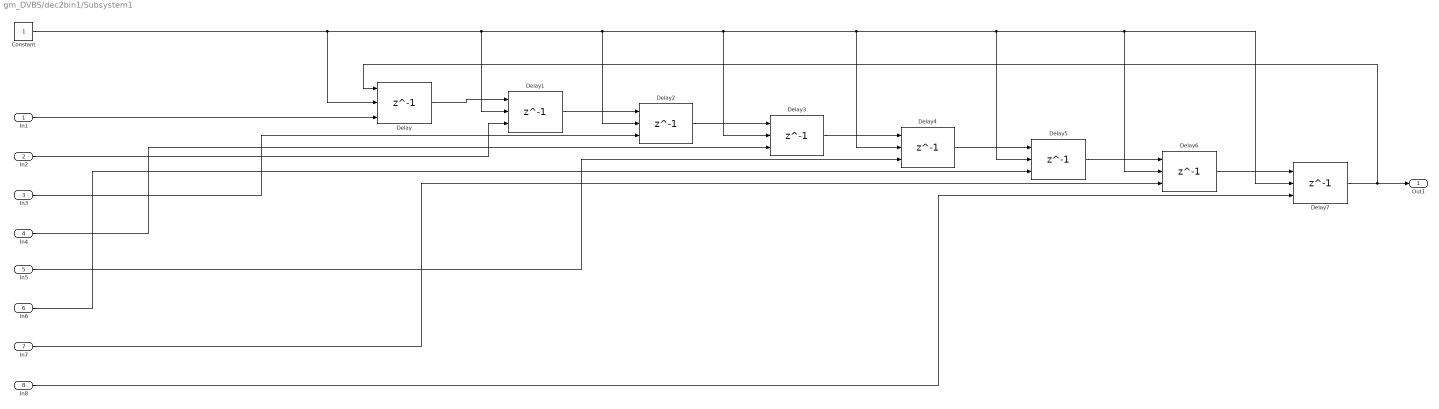
== system gm_DVBS/dec2bin1/Subsystem1 ==
  In1 : Inport
  In2 : Inport  Port=2
  In3 : Inport  Port=3
  In4 : Inport  Port=4
  In5 : Inport  Port=5
  In6 : Inport  Port=6
  In7 : Inport  Port=7
  In8 : Inport  Port=8
  Constant : Constant  OutDataTypeStr=boolean  SampleTime=1/rb
  Delay : Delay  DelayLength=1  InitialConditionSource=Input port  ExternalReset=Level hold
      settings: InputPortMap=u0,r5,p4
  Delay1 : Delay  DelayLength=1  InitialConditionSource=Input port  ExternalReset=Level hold
      settings: InputPortMap=u0,r5,p4
  Delay{2..7} (6 alike) : Delay  DelayLength=1  InitialConditionSource=Input port  ExternalReset=Rising
      settings: InputPortMap=u0,r5,p4
  Out1 : Outport
  wires:
  Constant/1 -> Delay6/2, Delay7/2, Delay5/2, Delay4/2, Delay3/2, Delay2/2, Delay1/2, Delay/2
  Delay7/1 -> Out1/1, Delay/1
  Delay3/1 -> Delay4/1
  Delay4/1 -> Delay5/1
  Delay5/1 -> Delay6/1
  Delay6/1 -> Delay7/1
  In6/1 -> Delay5/3
  In5/1 -> Delay4/3
  In8/1 -> Delay7/3
  In7/1 -> Delay6/3
  In4/1 -> Delay3/3
  In3/1 -> Delay2/3
  In2/1 -> Delay1/3
  In1/1 -> Delay/3
  Delay2/1 -> Delay3/1
  Delay1/1 -> Delay2/1
  Delay/1 -> Delay1/1

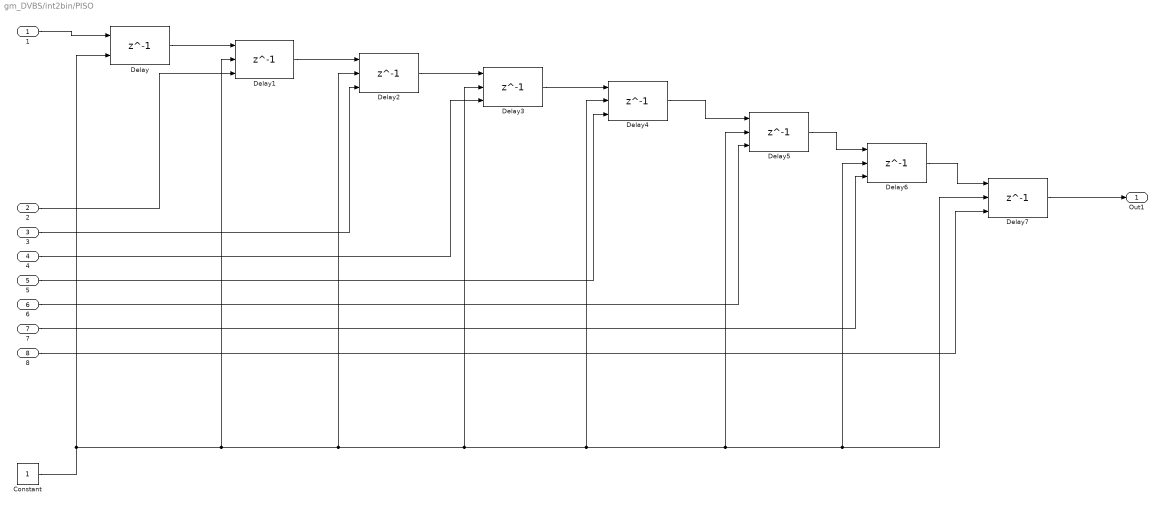
== system gm_DVBS/int2bin/PISO ==
  1 : Inport  OutDataTypeStr=boolean
  2 : Inport  Port=2
  3 : Inport  Port=3
  4 : Inport  Port=4
  5 : Inport  Port=5
  6 : Inport  Port=6
  7 : Inport  Port=7
  8 : Inport  Port=8
  Constant : Constant  OutDataTypeStr=boolean  SampleTime=1
  Delay : Delay  DelayLength=1  InitialCondition=0  ShowEnablePort=on  UseCircularBuffer=on  SampleTime=1
      settings: InputPortMap=u0,e6
  Delay{1..7} (7 alike) : Delay  DelayLength=1  InitialConditionSource=Input port  InitialCondition=0  ShowEnablePort=on  UseCircularBuffer=on  SampleTime=1
      settings: InputPortMap=u0,e6,p4
  Out1 : Outport
  wires:
  5/1 -> Delay4/3
  Delay7/1 -> Out1/1
  Delay6/1 -> Delay7/1
  6/1 -> Delay5/3
  8/1 -> Delay7/3
  7/1 -> Delay6/3
  Delay4/1 -> Delay5/1
  Delay5/1 -> Delay6/1
  Constant/1 -> Delay3/2, Delay7/2, Delay6/2, Delay5/2, Delay4/2, Delay2/2, Delay1/2, Delay/2
  Delay3/1 -> Delay4/1
  4/1 -> Delay3/3
  3/1 -> Delay2/3
  2/1 -> Delay1/3
  Delay2/1 -> Delay3/1
  Delay1/1 -> Delay2/1
  Delay/1 -> Delay1/1
  1/1 -> Delay/1

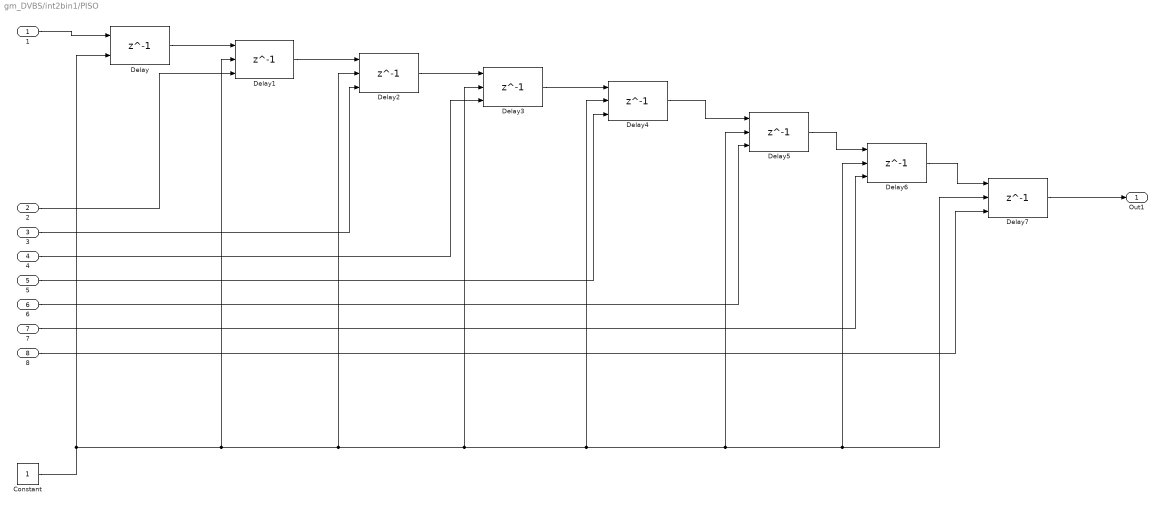
== system gm_DVBS/int2bin1/PISO ==
  1 : Inport  OutDataTypeStr=boolean
  2 : Inport  Port=2
  3 : Inport  Port=3
  4 : Inport  Port=4
  5 : Inport  Port=5
  6 : Inport  Port=6
  7 : Inport  Port=7
  8 : Inport  Port=8
  Constant : Constant  OutDataTypeStr=boolean  SampleTime=1
  Delay : Delay  DelayLength=1  InitialCondition=0  ShowEnablePort=on  UseCircularBuffer=on  SampleTime=1
      settings: InputPortMap=u0,e6
  Delay{1..7} (7 alike) : Delay  DelayLength=1  InitialConditionSource=Input port  InitialCondition=0  ShowEnablePort=on  UseCircularBuffer=on  SampleTime=1
      settings: InputPortMap=u0,e6,p4
  Out1 : Outport
  wires:
  5/1 -> Delay4/3
  Delay7/1 -> Out1/1
  Delay6/1 -> Delay7/1
  6/1 -> Delay5/3
  8/1 -> Delay7/3
  7/1 -> Delay6/3
  Delay4/1 -> Delay5/1
  Delay5/1 -> Delay6/1
  Constant/1 -> Delay3/2, Delay7/2, Delay6/2, Delay5/2, Delay4/2, Delay2/2, Delay1/2, Delay/2
  Delay3/1 -> Delay4/1
  4/1 -> Delay3/3
  3/1 -> Delay2/3
  2/1 -> Delay1/3
  Delay2/1 -> Delay3/1
  Delay1/1 -> Delay2/1
  Delay/1 -> Delay1/1
  1/1 -> Delay/1

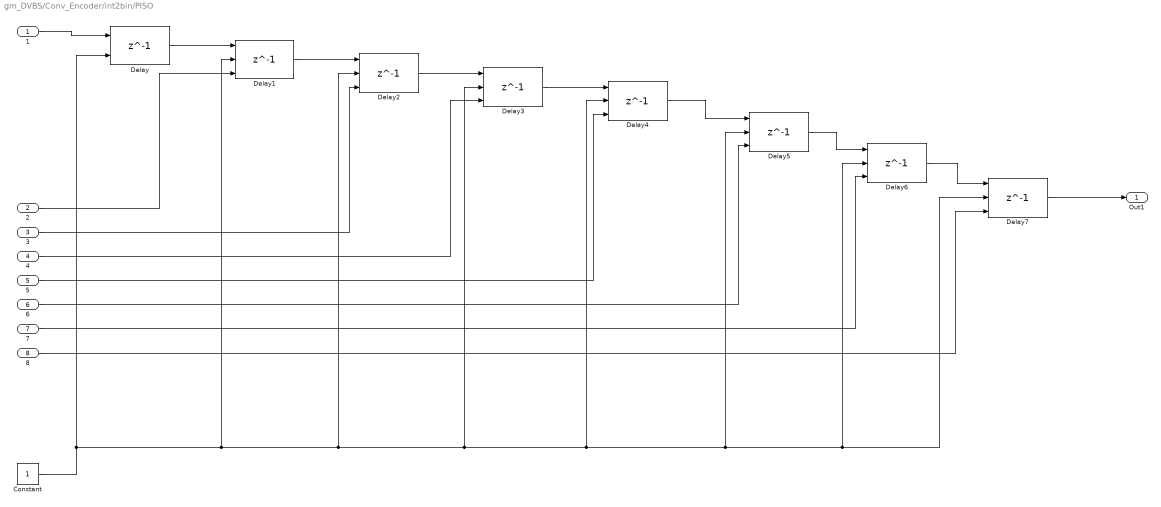
== system gm_DVBS/Conv_Encoder/int2bin/PISO ==
  1 : Inport
  2 : Inport  Port=2
  3 : Inport  Port=3
  4 : Inport  Port=4
  5 : Inport  Port=5
  6 : Inport  Port=6
  7 : Inport  Port=7
  8 : Inport  Port=8
  Constant : Constant  OutDataTypeStr=boolean  SampleTime=1
  Delay : Delay  DelayLength=1  InitialCondition=0  ShowEnablePort=on  UseCircularBuffer=on  SampleTime=1
      settings: InputPortMap=u0,e6
  Delay{1..7} (7 alike) : Delay  DelayLength=1  InitialConditionSource=Input port  InitialCondition=0  ShowEnablePort=on  UseCircularBuffer=on  SampleTime=1
      settings: InputPortMap=u0,e6,p4
  Out1 : Outport
  wires:
  5/1 -> Delay4/3
  Delay7/1 -> Out1/1
  Delay6/1 -> Delay7/1
  6/1 -> Delay5/3
  8/1 -> Delay7/3
  7/1 -> Delay6/3
  Delay4/1 -> Delay5/1
  Delay5/1 -> Delay6/1
  Constant/1 -> Delay3/2, Delay7/2, Delay6/2, Delay5/2, Delay4/2, Delay2/2, Delay1/2, Delay/2
  Delay3/1 -> Delay4/1
  4/1 -> Delay3/3
  3/1 -> Delay2/3
  2/1 -> Delay1/3
  Delay2/1 -> Delay3/1
  Delay1/1 -> Delay2/1
  Delay/1 -> Delay1/1
  1/1 -> Delay/1

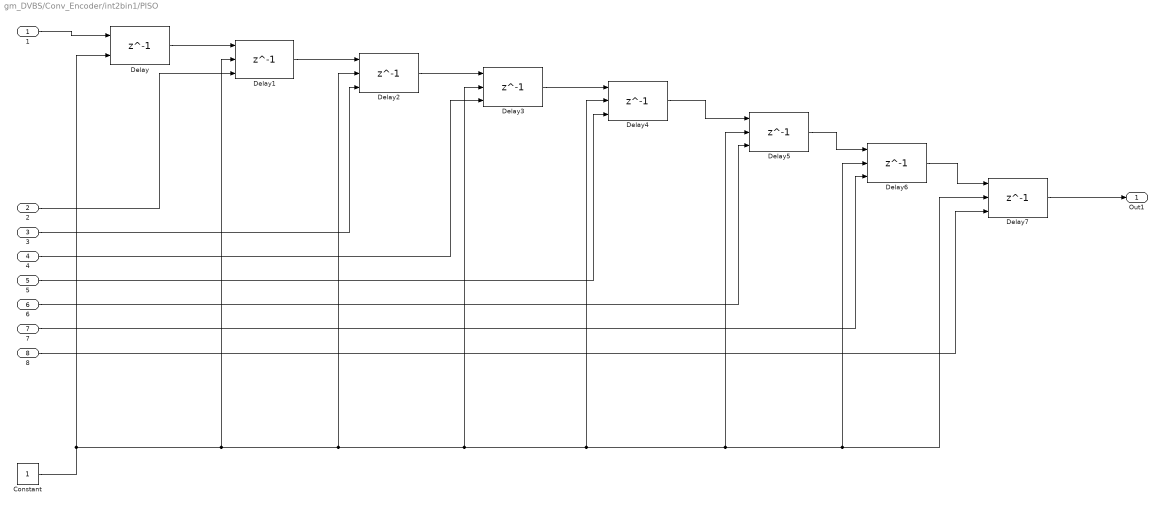
== system gm_DVBS/Conv_Encoder/int2bin1/PISO ==
  1 : Inport
  2 : Inport  Port=2
  3 : Inport  Port=3
  4 : Inport  Port=4
  5 : Inport  Port=5
  6 : Inport  Port=6
  7 : Inport  Port=7
  8 : Inport  Port=8
  Constant : Constant  OutDataTypeStr=boolean  SampleTime=1
  Delay : Delay  DelayLength=1  InitialCondition=0  ShowEnablePort=on  UseCircularBuffer=on  SampleTime=1
      settings: InputPortMap=u0,e6
  Delay{1..7} (7 alike) : Delay  DelayLength=1  InitialConditionSource=Input port  InitialCondition=0  ShowEnablePort=on  UseCircularBuffer=on  SampleTime=1
      settings: InputPortMap=u0,e6,p4
  Out1 : Outport
  wires:
  5/1 -> Delay4/3
  Delay7/1 -> Out1/1
  Delay6/1 -> Delay7/1
  6/1 -> Delay5/3
  8/1 -> Delay7/3
  7/1 -> Delay6/3
  Delay4/1 -> Delay5/1
  Delay5/1 -> Delay6/1
  Constant/1 -> Delay3/2, Delay7/2, Delay6/2, Delay5/2, Delay4/2, Delay2/2, Delay1/2, Delay/2
  Delay3/1 -> Delay4/1
  4/1 -> Delay3/3
  3/1 -> Delay2/3
  2/1 -> Delay1/3
  Delay2/1 -> Delay3/1
  Delay1/1 -> Delay2/1
  Delay/1 -> Delay1/1
  1/1 -> Delay/1

== matlab function gm_DVBS/Conv_Encoder/int2bin/uint8tobin ==
  data: input input; bitValue output
function bitValue = bitwiseOutput(input)
    % 逐bit输出输入数据的二进制表示
    bitValue=zeros(1,8);
    for i = 1:8
        bitValue(i) = bitget(input, i);
        
    end

end

== matlab function gm_DVBS/int2bin/uint8tobin ==
  data: input input; bitValue output
function bitValue = bitwiseOutput(input)
    % 逐bit输出输入数据的二进制表示
    bitValue=zeros(1,8);
    for i = 1:8
        bitValue(i) = bitget(input, i);
        
    end

end

== matlab function gm_DVBS/Subsystem/MATLAB Function ==
  data: dec_in input; bin_out output
function bin_out = fcn(dec_in)
%#codegen

bin_out=bitget(dec_in,8:-1:1);

== matlab function gm_DVBS/int2bin1/uint8tobin ==
  data: input input; bitValue output
function bitValue = bitwiseOutput(input)
    % 逐bit输出输入数据的二进制表示
    bitValue=zeros(1,8);
    for i = 1:8
        bitValue(i) = bitget(input, i);
        
    end

end

== matlab function gm_DVBS/Conv_Encoder/int2bin1/uint8tobin ==
  data: input input; bitValue output
function bitValue = bitwiseOutput(input)
    % 逐bit输出输入数据的二进制表示
    bitValue=zeros(1,8);
    for i = 1:8
        bitValue(i) = bitget(input, i);
        
    end

end
